simulink model "Model_1_0_legacy"  (R2017a)
settings: Solver=VariableStepAuto  StartTime=0.0  StopTime=1000  RelTol=1e-3
settings Model: Creator=Pål  LastModifiedBy=Pål
settings DataIOCC: ReturnWorkspaceOutputs=on
settings SFSimCC: SimUseLocalCustomCode=on
settings RTWCC: RTWUseLocalCustomCode=on

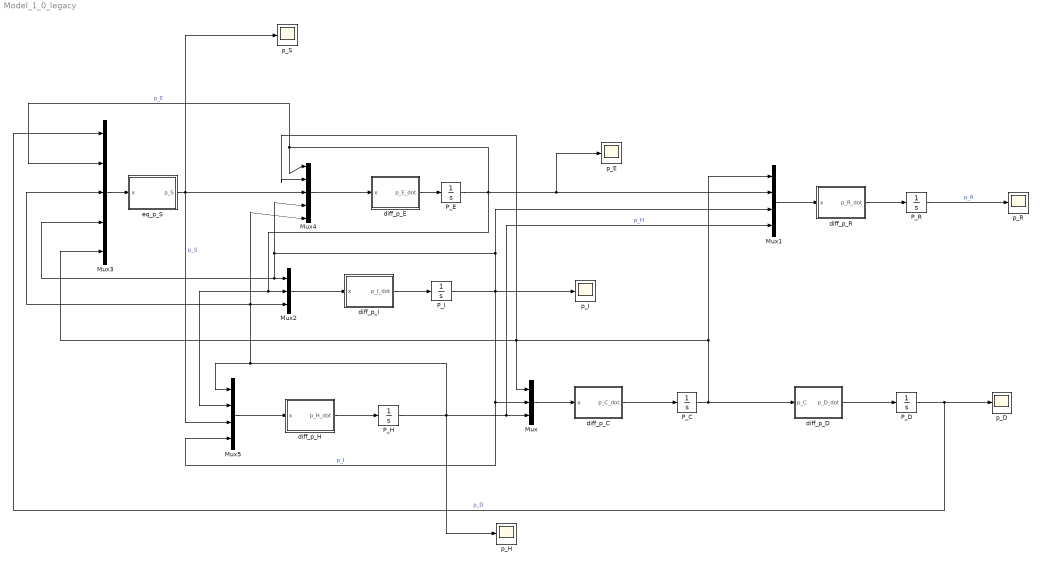
== system Model_1_0_legacy ==
  Mux : Mux  Inputs=3
  Mux1 : Mux
  Mux2 : Mux  Inputs=3
  Mux3 : Mux  Inputs=5
  Mux4 : Mux  Inputs=5
  Mux5 : Mux
  P_C : Integrator
  P_D : Integrator
  P_E : Integrator  InitialCondition=0.000025
  P_H : Integrator
  P_I : Integrator
  P_R : Integrator
  diff_p_C : MATLAB Function  TreatAsAtomicUnit=on
  diff_p_D : MATLAB Function  TreatAsAtomicUnit=on
  diff_p_E : MATLAB Function  TreatAsAtomicUnit=on
  diff_p_H : MATLAB Function  TreatAsAtomicUnit=on
  diff_p_I : MATLAB Function  TreatAsAtomicUnit=on
  diff_p_R : MATLAB Function  TreatAsAtomicUnit=on
  eq_p_S : MATLAB Function  TreatAsAtomicUnit=on
  p_D : Scope
  p_E : Scope
  p_H : Scope
  p_I : Scope
  p_R : Scope
  p_S : Scope
  wires:
  diff_p_C/1(p_C_dot) -> P_C/1
  diff_p_D/1(p_D_dot) -> P_D/1
  P_I/1 -> p_I/1, Mux3/4, Mux2/1, Mux4/4, Mux1/3, Mux5/4, Mux/2  "p_I"
  P_H/1 -> p_H/1, Mux5/1, Mux4/5, Mux3/3, Mux2/3, Mux1/4, Mux/3  "p_H"
  Mux/1 -> diff_p_C/1(x)
  diff_p_R/1(p_R_dot) -> P_R/1
  Mux1/1 -> diff_p_R/1(x)
  P_D/1 -> p_D/1, Mux3/1  "p_D"
  P_E/1 -> Mux5/2, Mux2/2, p_E/1, Mux1/2, Mux4/1, Mux3/2  "p_E"
  diff_p_H/1(p_H_dot) -> P_H/1
  diff_p_I/1(p_I_dot) -> P_I/1
  Mux2/1 -> diff_p_I/1(x)
  diff_p_E/1(p_E_dot) -> P_E/1
  Mux4/1 -> diff_p_E/1(x)
  Mux3/1 -> eq_p_S/1(x)
  P_C/1 -> Mux1/1, Mux/1, Mux4/2, Mux3/5, diff_p_D/1(p_C)
  Mux5/1 -> diff_p_H/1(x)
  P_R/1 -> p_R/1  "p_R"
  eq_p_S/1(p_S) -> p_S/1, Mux5/3, Mux4/3  "p_S"

== matlab function Model_1_0_legacy/diff_p_E ==
  data: x input double size=5; p_E_dot output double size=1
function p_E_dot = diff_p_E(x)
    model_1_0_param;
    p_E = x(1);
    p_C = x(2);
    p_S = x(3);
    p_I = x(4);
    p_H = x(5);
    
    p_E_dot = (beta_E*p_E + beta_H*p_H + beta_I*p_I + beta_C*p_C)*p_S ...
              - eta*p_E - (alpha_E + delta_E)*p_E + gamma_E*p_H;
end

== matlab function Model_1_0_legacy/eq_p_S ==
  data: x input double size=5; p_S output double size=1
function p_S = eq_p_S(x)
    model_1_0_param;
    p_D = x(1);
    p_E = x(2);
    p_H = x(3);
    p_I = x(4);
    p_C = x(5);
    
    
    p_S = 1 - p_D - p_E - p_H - p_I - p_C;
end

== matlab function Model_1_0_legacy/diff_p_I ==
  data: x input double size=3; p_I_dot output double size=1
function p_I_dot = diff_p_I(x)
    model_1_0_param;
    p_I = x(1);
    p_E = x(2);
    p_H = x(3);

    p_I_dot = eta*p_E - (alpha_I + xi + delta_I)*p_I + gamma_I*p_H;
end

== matlab function Model_1_0_legacy/diff_p_R ==
  data: x input double size=4; p_R_dot output double size=1
function p_R_dot = diff_p_R(x)
    model_1_0_param;
    p_C = x(1);
    p_E = x(2);
    p_I = x(3);
    p_H = x(4);
    
    p_R_dot = alpha_E*p_E + alpha_I*p_I + gamma_R*p_H + rho*p_C;
end

== matlab function Model_1_0_legacy/diff_p_D ==
  data: p_C input size=1; p_D_dot output size=1
function p_D_dot = diff_p_D(p_C)
    model_1_0_param;
    p_D_dot = mu*p_C;
end

== matlab function Model_1_0_legacy/diff_p_H ==
  data: x input size=4; p_H_dot output size=1
function p_H_dot = diff_p_H(x)
    model_1_0_param;
    p_H = x(1);
    p_E = x(2);
    p_S = x(3);
    p_I = x(4);
    
    p_H_dot = delta_S*p_S + delta_E*p_E + delta_I*p_I - ...
              (gamma_S + gamma_E + gamma_I + gamma_R + gamma_C) * p_H;
end

== matlab function Model_1_0_legacy/diff_p_C ==
  data: x input size=3; p_C_dot output size=1
function p_C_dot = diff_p_C(x)
    model_1_0_param;
    p_C = x(1);
    p_I = x(2);
    p_H = x(3);

    p_C_dot = xi*p_I + gamma_C*p_H - (rho + mu)*p_C;
end
